simulink library "RealTimeLibrary"  (R2016b)
settings: Solver=ode45  StartTime=0.0  StopTime=10.0  RelTol=1e-3  EnableMultiTasking=on
undefined symbols (not defined in the file): CassieParameters, motor, pelvisMedulla
libraries: xpcethercatlib x75, simulink x1
settings Model: Creator=Mikhail  LastModifiedBy=Mikhail
settings DataIOCC: LimitDataPoints=on
settings OptimizationCC: LifeSpan=inf
settings DebuggingCC: AllowSymbolicDim=off  SFUnexpectedBacktrackingDiag=warning  SFNoUnconditionalDefaultTransitionDiag=warning  SFExecutionAtInitializationDiag=none
settings GRTTargetCC: TargetLangStandard=C89/C90 (ANSI)  GeneratePreprocessorConditionals=Disable all
settings ConfigComp: CovMetricSettings=dw  CovHtmlReporting=on  CovSaveCumulativeToWorkspaceVar=on  CovSaveSingleToWorkspaceVar=on  CovExternalEMLEnable=off

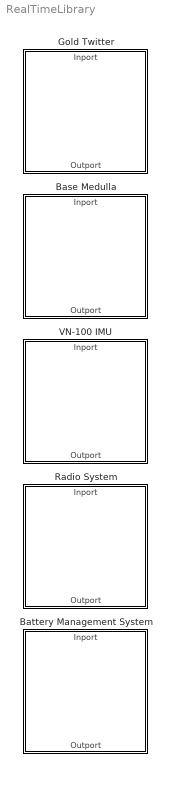
== system RealTimeLibrary ==
  Base Medulla : Subsystem  mask{structureName='pelvisMedulla', ethercatName='Pelvis Medulla'}
      mask prompts: structureName "Structure Name"; ethercatName "EtherCAT Name"
      mask init:
      | % Set bus assignments
      | set_param([gcb '/Base Inputs Bus Assignment'], ...
      |   'AssignedSignals', [...
      |     structureName '.baseInputs.cpuLoad,', ...
      |     structureName '.baseInputs.counter']);
      | 
      | % Set PDO recieve signal names
      | set_param([gcb '/CPU Load PDO Receive'], ...
      |   'sig_name', [ethercatName '.Base Inputs.CPU Load']);
      | set_param([gcb '/Counter PDO Receive'], ...
      |   'sig_name', [ethercatName '.Base Inputs.Counter']);
      mask Display: image('Medulla.png');
  Battery Management System : Subsystem
      mask Display: image('BQ76PL536A.png');
  Gold Twitter : Subsystem  mask{structureName='motor', ethercatName='Drive (Elmo Drive)', gearRatio=1, torqueConstant=1, encoderCounts=2^13, peakCurrentLimit=50}
      mask prompts: structureName "Structure Name"; ethercatName "EtherCAT Name"; gearRatio "Gear Ratio"; torqueConstant "Torque Constant"; encoderCounts "Encoder Counts"; peakCurrentLimit "Peak Current Limit"
      mask init:
      | % Set bus selectors
      | set_param([gcb '/Target Torque Bus Selector'], ...
      |   'OutputSignals', [structureName '.outputs.torque']);
      | set_param([gcb '/Status Word Bus Selector'], ...
      |   'OutputSignals', [structureName '.inputs.statusWord']);
      | 
      | % Set bus assignment
      | set_param([gcb '/Gold Twitter Bus Assignment'], ...
      |   'AssignedSignals', [...
      |     structureName '.inputs.statusWord,', ...
      |     structureName '.inputs.position,', ...
      |     structureName '.inputs.torque,', ...
      |     structureName '.inputs.amplifierTemperature,', ...
      |     structureName '.inputs.statorTemperature']);
      | 
      | % Set PDO transmit
      | set_param([gcb '/Mode of Operation PDO Transmit'], ...
      |   'sig_name', [ethercatName '.Outputs.Mode of operation']);
      | set_param([gcb '/Target Torque PDO Transmit'], ...
      |   'sig_name', [ethercatName '.Outputs.Target Torque']);
      | set_param([gcb '/Control Word PDO Transmit'], ...
      |   'sig_name', [ethercatName '.Outputs.Control word']);
      | 
      | % Set PDO receive
      | set_param([gcb '/Status Word PDO Receive'], ...
      |   'sig_name', [ethercatName '.Inputs.Status word']);
      | set_param([gcb '/Position PDO Receive'], ...
      |   'sig_name', [ethercatName '.Inputs.Position actual value']);
      | set_param([gcb '/Torque PDO Receive'], ...
      |   'sig_name', [ethercatName '.Inputs.Torque actual value']);
      | set_param([gcb '/Stator Temperature PDO Receive'], ...
      |   'sig_name', [ethercatName '.Inputs.Stator Temp']);
      | 
      | % Set SDO upload
      | set_param([gcb '/Amplifier Temperature Async SDO Upload'], ...
      |   'index', '8867');
      | set_param([gcb '/Amplifier Temperature Async SDO Upload'], ...
      |   'subIndex', '1');
      | set_param([gcb '/Amplifier Temperature Async SDO Upload'], ...
      |   'slave_name', ethercatName);
      mask Display: image('Gold Twitter.png')
  Radio System : Subsystem
      mask Display: image('Fr Sky Taranis.png');
  VN-100 IMU : Subsystem
      mask Display: image('VN-100 IMU.png');

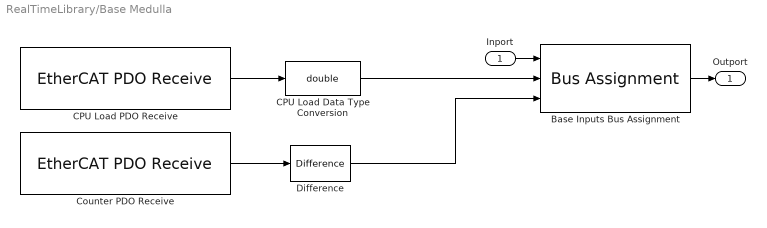
== system RealTimeLibrary/Base Medulla ==
  Inport : Inport  OutDataTypeStr=Bus: cassieEtherCATBus  SampleTime=CassieParameters.etherCATSampleTime
  Base Inputs Bus Assignment : BusAssignment  AssignedSignals=pelvisMedulla.baseInputs.cpuLoad,pelvisMedulla.baseInputs.counter
  CPU Load Data Type Conversion : DataTypeConversion  OutDataTypeStr=double
  CPU Load PDO Receive : xpcethercatlib/EtherCAT PDO Receive  Priority=2  sig_name=Pelvis Medulla.Base Inputs.CPU Load  sig_offset=600  sig_type=uint16  type_size=16  sig_dim=1  device_id=0  sample_time=0.000500
  Counter PDO Receive : xpcethercatlib/EtherCAT PDO Receive  Priority=2  sig_name=Pelvis Medulla.Base Inputs.Counter  sig_offset=592  sig_type=uint8  type_size=8  sig_dim=1  device_id=0  sample_time=0.000500
  Difference : simulink/Discrete/Difference  ICPrevInput=0.0  OutMin=[]  OutMax=[]  OutDataType=fixdt(1, 16)  OutScaling=2^-10  DoSatur=off
  Outport : Outport  OutDataTypeStr=Bus: cassieEtherCATBus  SampleTime=CassieParameters.etherCATSampleTime
  wires:
  Base Inputs Bus Assignment/1 -> Outport/1
  Counter PDO Receive/1 -> Difference/1
  Difference/1 -> Base Inputs Bus Assignment/3
  Inport/1 -> Base Inputs Bus Assignment/1
  CPU Load PDO Receive/1 -> CPU Load Data Type Conversion/1
  CPU Load Data Type Conversion/1 -> Base Inputs Bus Assignment/2

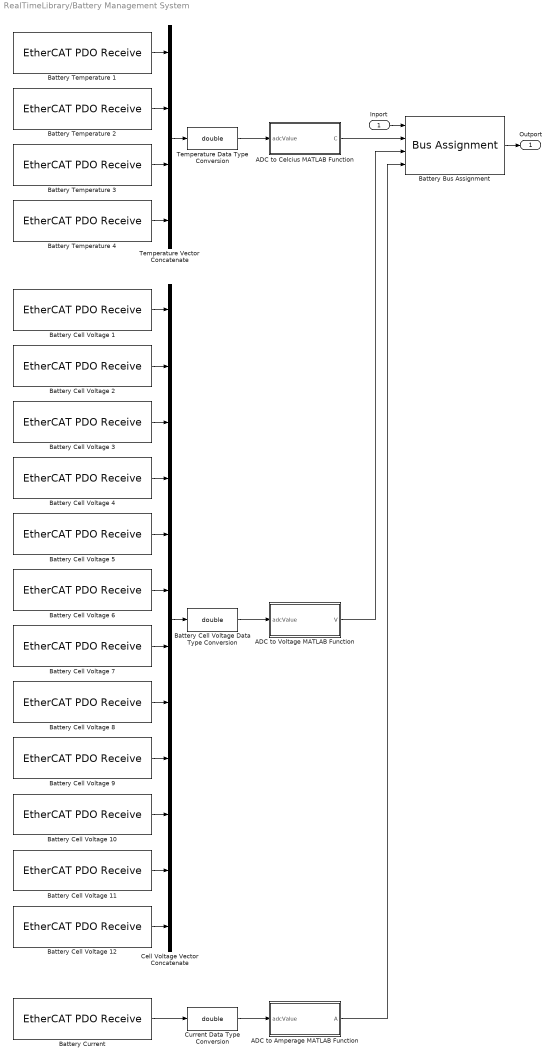
== system RealTimeLibrary/Battery Management System ==
  Inport : Inport  OutDataTypeStr=Bus: cassieEtherCATBus  SampleTime=CassieParameters.etherCATSampleTime
  ADC to Amperage MATLAB Function : MATLAB Function  TreatAsAtomicUnit=on
  ADC to Celcius MATLAB Function : MATLAB Function  TreatAsAtomicUnit=on
  ADC to Voltage MATLAB Function : MATLAB Function  TreatAsAtomicUnit=on
  Battery Bus Assignment : BusAssignment  AssignedSignals=pelvisMedulla.inputs.batteryTemperature,pelvisMedulla.inputs.batteryCellVoltage,pelvisMedulla.inputs.batteryCurrent
  Battery Cell Voltage Data Type Conversion : DataTypeConversion  OutDataTypeStr=double
  Battery Cell Voltage 1 : xpcethercatlib/EtherCAT PDO Receive  Priority=2  sig_name=Pelvis Medulla.BMS Inputs.Cell Voltage 01  sig_offset=1528  sig_type=uint16  type_size=16  sig_dim=1  device_id=0  sample_time=0.000500
  Battery Cell Voltage 10 : xpcethercatlib/EtherCAT PDO Receive  Priority=2  sig_name=Pelvis Medulla.BMS Inputs.Cell Voltage 10  sig_offset=1672  sig_type=uint16  type_size=16  sig_dim=1  device_id=0  sample_time=0.000500
  Battery Cell Voltage 11 : xpcethercatlib/EtherCAT PDO Receive  Priority=2  sig_name=Pelvis Medulla.BMS Inputs.Cell Voltage 11  sig_offset=1688  sig_type=uint16  type_size=16  sig_dim=1  device_id=0  sample_time=0.000500
  Battery Cell Voltage 12 : xpcethercatlib/EtherCAT PDO Receive  Priority=2  sig_name=Pelvis Medulla.BMS Inputs.Cell Voltage 12  sig_offset=1704  sig_type=uint16  type_size=16  sig_dim=1  device_id=0  sample_time=0.000500
  Battery Cell Voltage 2 : xpcethercatlib/EtherCAT PDO Receive  Priority=2  sig_name=Pelvis Medulla.BMS Inputs.Cell Voltage 02  sig_offset=1544  sig_type=uint16  type_size=16  sig_dim=1  device_id=0  sample_time=0.000500
  Battery Cell Voltage 3 : xpcethercatlib/EtherCAT PDO Receive  Priority=2  sig_name=Pelvis Medulla.BMS Inputs.Cell Voltage 03  sig_offset=1560  sig_type=uint16  type_size=16  sig_dim=1  device_id=0  sample_time=0.000500
  Battery Cell Voltage 4 : xpcethercatlib/EtherCAT PDO Receive  Priority=2  sig_name=Pelvis Medulla.BMS Inputs.Cell Voltage 04  sig_offset=1576  sig_type=uint16  type_size=16  sig_dim=1  device_id=0  sample_time=0.000500
  Battery Cell Voltage 5 : xpcethercatlib/EtherCAT PDO Receive  Priority=2  sig_name=Pelvis Medulla.BMS Inputs.Cell Voltage 05  sig_offset=1592  sig_type=uint16  type_size=16  sig_dim=1  device_id=0  sample_time=0.000500
  Battery Cell Voltage 6 : xpcethercatlib/EtherCAT PDO Receive  Priority=2  sig_name=Pelvis Medulla.BMS Inputs.Cell Voltage 06  sig_offset=1608  sig_type=uint16  type_size=16  sig_dim=1  device_id=0  sample_time=0.000500
  Battery Cell Voltage 7 : xpcethercatlib/EtherCAT PDO Receive  Priority=2  sig_name=Pelvis Medulla.BMS Inputs.Cell Voltage 07  sig_offset=1624  sig_type=uint16  type_size=16  sig_dim=1  device_id=0  sample_time=0.000500
  Battery Cell Voltage 8 : xpcethercatlib/EtherCAT PDO Receive  Priority=2  sig_name=Pelvis Medulla.BMS Inputs.Cell Voltage 08  sig_offset=1640  sig_type=uint16  type_size=16  sig_dim=1  device_id=0  sample_time=0.000500
  Battery Cell Voltage 9 : xpcethercatlib/EtherCAT PDO Receive  Priority=2  sig_name=Pelvis Medulla.BMS Inputs.Cell Voltage 09  sig_offset=1656  sig_type=uint16  type_size=16  sig_dim=1  device_id=0  sample_time=0.000500
  Battery Current : xpcethercatlib/EtherCAT PDO Receive  Priority=2  sig_name=Pelvis Medulla.BMS Inputs.Current  sig_offset=1784  sig_type=uint16  type_size=16  sig_dim=1  device_id=0  sample_time=0.000500
  Battery Temperature 1 : xpcethercatlib/EtherCAT PDO Receive  Priority=2  sig_name=Pelvis Medulla.BMS Inputs.Temperature 1  sig_offset=1720  sig_type=uint16  type_size=16  sig_dim=1  device_id=0  sample_time=0.000500
  Battery Temperature 2 : xpcethercatlib/EtherCAT PDO Receive  Priority=2  sig_name=Pelvis Medulla.BMS Inputs.Temperature 2  sig_offset=1736  sig_type=uint16  type_size=16  sig_dim=1  device_id=0  sample_time=0.000500
  Battery Temperature 3 : xpcethercatlib/EtherCAT PDO Receive  Priority=2  sig_name=Pelvis Medulla.BMS Inputs.Temperature 3  sig_offset=1752  sig_type=uint16  type_size=16  sig_dim=1  device_id=0  sample_time=0.000500
  Battery Temperature 4 : xpcethercatlib/EtherCAT PDO Receive  Priority=2  sig_name=Pelvis Medulla.BMS Inputs.Temperature 4  sig_offset=1768  sig_type=uint16  type_size=16  sig_dim=1  device_id=0  sample_time=0.000500
  Cell Voltage Vector Concatenate : Concatenate  NumInputs=12
  Current Data Type Conversion : DataTypeConversion  OutDataTypeStr=double
  Temperature Data Type Conversion : DataTypeConversion  OutDataTypeStr=double
  Temperature Vector Concatenate : Concatenate  NumInputs=4
  Outport : Outport  OutDataTypeStr=Bus: cassieEtherCATBus  SampleTime=CassieParameters.etherCATSampleTime
  wires:
  Battery Temperature 1/1 -> Temperature Vector Concatenate/1
  Battery Temperature 2/1 -> Temperature Vector Concatenate/2
  Battery Temperature 3/1 -> Temperature Vector Concatenate/3
  Battery Temperature 4/1 -> Temperature Vector Concatenate/4
  Battery Cell Voltage 1/1 -> Cell Voltage Vector Concatenate/1
  Battery Cell Voltage 2/1 -> Cell Voltage Vector Concatenate/2
  Battery Cell Voltage 3/1 -> Cell Voltage Vector Concatenate/3
  Battery Cell Voltage 4/1 -> Cell Voltage Vector Concatenate/4
  Battery Cell Voltage 5/1 -> Cell Voltage Vector Concatenate/5
  Battery Cell Voltage 6/1 -> Cell Voltage Vector Concatenate/6
  Battery Cell Voltage 7/1 -> Cell Voltage Vector Concatenate/7
  Battery Cell Voltage 8/1 -> Cell Voltage Vector Concatenate/8
  Battery Cell Voltage 9/1 -> Cell Voltage Vector Concatenate/9
  Battery Cell Voltage 10/1 -> Cell Voltage Vector Concatenate/10
  Battery Cell Voltage 11/1 -> Cell Voltage Vector Concatenate/11
  Battery Cell Voltage 12/1 -> Cell Voltage Vector Concatenate/12
  Temperature Vector Concatenate/1 -> Temperature Data Type Conversion/1
  Cell Voltage Vector Concatenate/1 -> Battery Cell Voltage Data Type Conversion/1
  ADC to Voltage MATLAB Function/1(V) -> Battery Bus Assignment/3
  Battery Current/1 -> Current Data Type Conversion/1
  ADC to Celcius MATLAB Function/1(C) -> Battery Bus Assignment/2
  Battery Bus Assignment/1 -> Outport/1
  Inport/1 -> Battery Bus Assignment/1
  Temperature Data Type Conversion/1 -> ADC to Celcius MATLAB Function/1(adcValue)
  Battery Cell Voltage Data Type Conversion/1 -> ADC to Voltage MATLAB Function/1(adcValue)
  ADC to Amperage MATLAB Function/1(A) -> Battery Bus Assignment/4
  Current Data Type Conversion/1 -> ADC to Amperage MATLAB Function/1(adcValue)

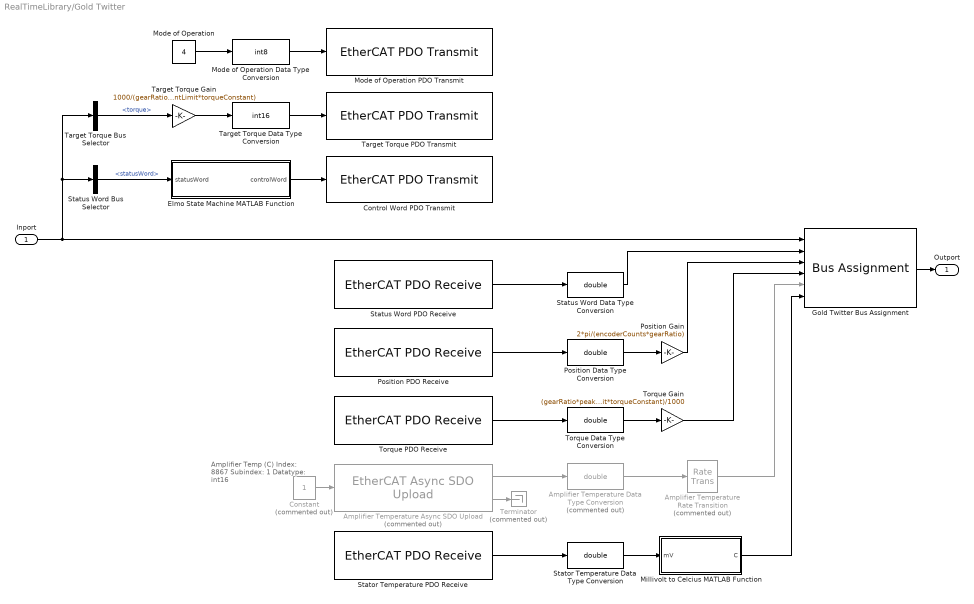
== system RealTimeLibrary/Gold Twitter ==
  note: Amplifier Temp (C)
      | Index: 8867
      | Subindex: 1
      | Datatype: int16
  Inport : Inport  PortDimensions=1
  Amplifier Temperature Data Type Conversion : DataTypeConversion  Commented=on  OutDataTypeStr=double
  Amplifier Temperature Rate Transition : RateTransition  Commented=on
  Amplifier Temperature Async SDO Upload : xpcethercatlib/EtherCAT Async SDO Upload  Commented=on  index=8867  subIndex=1  sig_type=int16  sig_dim=1  device_id=0  slave_name=Drive (Elmo Drive)  sample_time=1/100  slave_addr=0  selected_slave=Term 1 (EK1100)  timeout=500  slave_found=0
  Constant : Constant  Commented=on  OutDataTypeStr=int32
  Control Word PDO Transmit : xpcethercatlib/EtherCAT PDO Transmit   Priority=3  sig_name=Drive (Elmo Drive).Outputs.Control word  sig_offset=2144  sig_type=uint16  type_size=16  sig_dim=1  device_id=0  sample_time=0.001000
  Elmo State Machine MATLAB Function : MATLAB Function  TreatAsAtomicUnit=on
  Gold Twitter Bus Assignment : BusAssignment  AssignedSignals=motor.inputs.statusWord,motor.inputs.position,motor.inputs.torque,motor.inputs.amplifierTemperature,motor.inputs.statorTemperature
  Millivolt to Celcius MATLAB Function : MATLAB Function  TreatAsAtomicUnit=on
  Mode of Operation : Constant  Value=4  OutDataTypeStr=Inherit: Inherit via back propagation
  Mode of Operation Data Type Conversion : DataTypeConversion  OutDataTypeStr=int8
  Mode of Operation PDO Transmit : xpcethercatlib/EtherCAT PDO Transmit   Priority=3  sig_name=Drive (Elmo Drive).Outputs.Mode of operation  sig_offset=2160  sig_type=int8  type_size=8  sig_dim=1  device_id=0  sample_time=0.001000
  Position Data Type Conversion : DataTypeConversion  OutDataTypeStr=double
  Position Gain : Gain  Gain=2*pi/(encoderCounts*gearRatio)
  Position PDO Receive : xpcethercatlib/EtherCAT PDO Receive  Priority=2  sig_name=Drive (Elmo Drive).Inputs.Position actual value  sig_offset=2128  sig_type=int32  type_size=32  sig_dim=1  device_id=0  sample_time=0.001000
  Stator Temperature Data Type Conversion : DataTypeConversion  OutDataTypeStr=double
  Stator Temperature PDO Receive : xpcethercatlib/EtherCAT PDO Receive  Priority=2  sig_name=Drive (Elmo Drive).Inputs.Stator Temp  sig_offset=2128  sig_type=int32  type_size=32  sig_dim=1  device_id=0  sample_time=0.001000
  Status Word Bus Selector : BusSelector  OutputSignals=motor.inputs.statusWord
  Status Word Data Type Conversion : DataTypeConversion  OutDataTypeStr=double
  Status Word PDO Receive : xpcethercatlib/EtherCAT PDO Receive  Priority=2  sig_name=Drive (Elmo Drive).Inputs.Status word  sig_offset=2176  sig_type=uint16  type_size=16  sig_dim=1  device_id=0  sample_time=0.001000
  Target Torque Bus Selector : BusSelector  OutputSignals=motor.outputs.torque
  Target Torque Data Type Conversion : DataTypeConversion  OutDataTypeStr=int16
  Target Torque Gain : Gain  Gain=1000/(gearRatio*peakCurrentLimit*torqueConstant)
  Target Torque PDO Transmit : xpcethercatlib/EtherCAT PDO Transmit   Priority=3  sig_name=Drive (Elmo Drive).Outputs.Target Torque  sig_offset=2128  sig_type=int16  type_size=16  sig_dim=1  device_id=0  sample_time=0.001000
  Terminator : Terminator  Commented=on
  Torque Data Type Conversion : DataTypeConversion  OutDataTypeStr=double
  Torque Gain : Gain  Gain=(gearRatio*peakCurrentLimit*torqueConstant)/1000
  Torque PDO Receive : xpcethercatlib/EtherCAT PDO Receive  Priority=2  sig_name=Drive (Elmo Drive).Inputs.Torque actual value  sig_offset=2128  sig_type=int32  type_size=32  sig_dim=1  device_id=0  sample_time=0.001000
  Outport : Outport  PortDimensions=1
  wires:
  Status Word Data Type Conversion/1 -> Gold Twitter Bus Assignment/2
  Position Data Type Conversion/1 -> Position Gain/1
  Target Torque Bus Selector/1 -> Target Torque Gain/1  "<torque>"
  Gold Twitter Bus Assignment/1 -> Outport/1
  Target Torque Gain/1 -> Target Torque Data Type Conversion/1
  Position PDO Receive/1 -> Position Data Type Conversion/1
  Target Torque Data Type Conversion/1 -> Target Torque PDO Transmit/1
  Mode of Operation Data Type Conversion/1 -> Mode of Operation PDO Transmit/1
  Mode of Operation/1 -> Mode of Operation Data Type Conversion/1
  Status Word PDO Receive/1 -> Status Word Data Type Conversion/1
  Elmo State Machine MATLAB Function/1(controlWord) -> Control Word PDO Transmit/1
  Inport/1 -> Status Word Bus Selector/1, Target Torque Bus Selector/1, Gold Twitter Bus Assignment/1
  Status Word Bus Selector/1 -> Elmo State Machine MATLAB Function/1(statusWord)  "<statusWord>"
  Torque Data Type Conversion/1 -> Torque Gain/1
  Torque PDO Receive/1 -> Torque Data Type Conversion/1
  Position Gain/1 -> Gold Twitter Bus Assignment/3
  Torque Gain/1 -> Gold Twitter Bus Assignment/4
  Constant/1 -> Amplifier Temperature Async SDO Upload/1
  Amplifier Temperature Async SDO Upload/1 -> Amplifier Temperature Data Type Conversion/1
  Amplifier Temperature Async SDO Upload/2 -> Terminator/1
  Stator Temperature Data Type Conversion/1 -> Millivolt to Celcius MATLAB Function/1(mV)
  Stator Temperature PDO Receive/1 -> Stator Temperature Data Type Conversion/1
  Amplifier Temperature Data Type Conversion/1 -> Amplifier Temperature Rate Transition/1
  Millivolt to Celcius MATLAB Function/1(C) -> Gold Twitter Bus Assignment/6
  Amplifier Temperature Rate Transition/1 -> Gold Twitter Bus Assignment/5

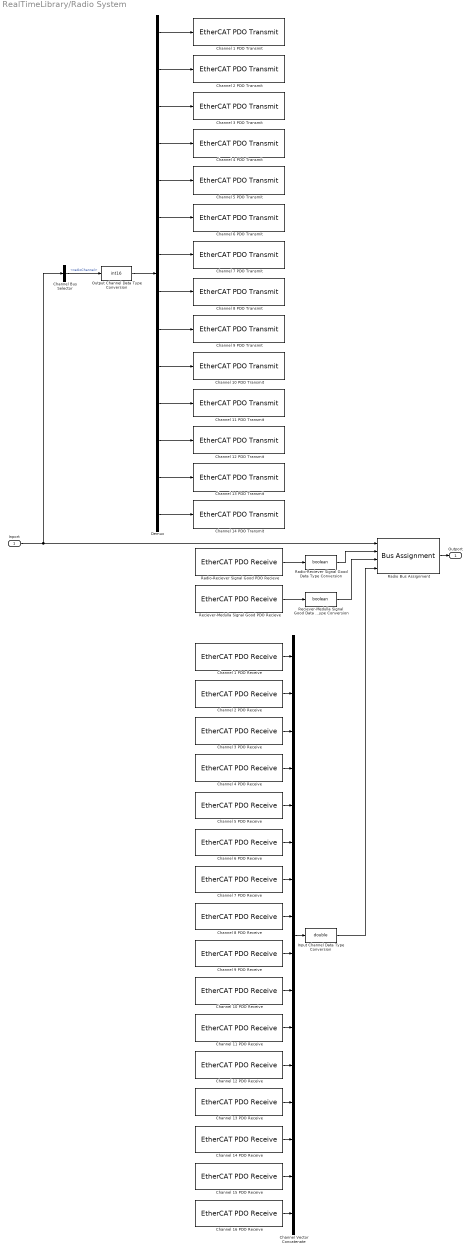
== system RealTimeLibrary/Radio System ==
  Inport : Inport  OutDataTypeStr=Bus: cassieEtherCATBus  SampleTime=CassieParameters.etherCATSampleTime
  Channel Bus Selector : BusSelector  OutputSignals=pelvisMedulla.outputs.radioChannel
  Channel Vector Concatenate : Concatenate  NumInputs=16
  Channel 1 PDO Receive : xpcethercatlib/EtherCAT PDO Receive  Priority=2  sig_name=Pelvis Medulla.Radio Inputs.Channel 01  sig_offset=616  sig_type=int16  type_size=16  sig_dim=1  device_id=0  sample_time=0.000500
  Channel 1 PDO Transmit : xpcethercatlib/EtherCAT PDO Transmit   Priority=3  sig_name=Pelvis Medulla.Radio Outputs.Channel 01  sig_offset=592  sig_type=int16  type_size=16  sig_dim=1  device_id=0  sample_time=0.000500
  Channel 10 PDO Receive : xpcethercatlib/EtherCAT PDO Receive  Priority=2  sig_name=Pelvis Medulla.Radio Inputs.Channel 10  sig_offset=760  sig_type=int16  type_size=16  sig_dim=1  device_id=0  sample_time=0.000500
  Channel 10 PDO Transmit : xpcethercatlib/EtherCAT PDO Transmit   Priority=3  sig_name=Pelvis Medulla.Radio Outputs.Channel 10  sig_offset=736  sig_type=int16  type_size=16  sig_dim=1  device_id=0  sample_time=0.000500
  Channel 11 PDO Receive : xpcethercatlib/EtherCAT PDO Receive  Priority=2  sig_name=Pelvis Medulla.Radio Inputs.Channel 11  sig_offset=776  sig_type=int16  type_size=16  sig_dim=1  device_id=0  sample_time=0.000500
  Channel 11 PDO Transmit : xpcethercatlib/EtherCAT PDO Transmit   Priority=3  sig_name=Pelvis Medulla.Radio Outputs.Channel 11  sig_offset=752  sig_type=int16  type_size=16  sig_dim=1  device_id=0  sample_time=0.000500
  Channel 12 PDO Receive : xpcethercatlib/EtherCAT PDO Receive  Priority=2  sig_name=Pelvis Medulla.Radio Inputs.Channel 12  sig_offset=792  sig_type=int16  type_size=16  sig_dim=1  device_id=0  sample_time=0.000500
  Channel 12 PDO Transmit : xpcethercatlib/EtherCAT PDO Transmit   Priority=3  sig_name=Pelvis Medulla.Radio Outputs.Channel 12  sig_offset=768  sig_type=int16  type_size=16  sig_dim=1  device_id=0  sample_time=0.000500
  Channel 13 PDO Receive : xpcethercatlib/EtherCAT PDO Receive  Priority=2  sig_name=Pelvis Medulla.Radio Inputs.Channel 13  sig_offset=808  sig_type=int16  type_size=16  sig_dim=1  device_id=0  sample_time=0.000500
  Channel 13 PDO Transmit : xpcethercatlib/EtherCAT PDO Transmit   Priority=3  sig_name=Pelvis Medulla.Radio Outputs.Channel 13  sig_offset=784  sig_type=int16  type_size=16  sig_dim=1  device_id=0  sample_time=0.000500
  Channel 14 PDO Receive : xpcethercatlib/EtherCAT PDO Receive  Priority=2  sig_name=Pelvis Medulla.Radio Inputs.Channel 14  sig_offset=824  sig_type=int16  type_size=16  sig_dim=1  device_id=0  sample_time=0.000500
  Channel 14 PDO Transmit : xpcethercatlib/EtherCAT PDO Transmit   Priority=3  sig_name=Pelvis Medulla.Radio Outputs.Channel 14  sig_offset=800  sig_type=int16  type_size=16  sig_dim=1  device_id=0  sample_time=0.000500
  Channel 15 PDO Receive : xpcethercatlib/EtherCAT PDO Receive  Priority=2  sig_name=Pelvis Medulla.Radio Inputs.Channel 15  sig_offset=840  sig_type=int16  type_size=16  sig_dim=1  device_id=0  sample_time=0.000500
  Channel 16 PDO Receive : xpcethercatlib/EtherCAT PDO Receive  Priority=2  sig_name=Pelvis Medulla.Radio Inputs.Channel 16  sig_offset=856  sig_type=int16  type_size=16  sig_dim=1  device_id=0  sample_time=0.000500
  Channel 2 PDO Receive : xpcethercatlib/EtherCAT PDO Receive  Priority=2  sig_name=Pelvis Medulla.Radio Inputs.Channel 02  sig_offset=632  sig_type=int16  type_size=16  sig_dim=1  device_id=0  sample_time=0.000500
  Channel 2 PDO Transmit : xpcethercatlib/EtherCAT PDO Transmit   Priority=3  sig_name=Pelvis Medulla.Radio Outputs.Channel 02  sig_offset=608  sig_type=int16  type_size=16  sig_dim=1  device_id=0  sample_time=0.000500
  Channel 3 PDO Receive : xpcethercatlib/EtherCAT PDO Receive  Priority=2  sig_name=Pelvis Medulla.Radio Inputs.Channel 03  sig_offset=648  sig_type=int16  type_size=16  sig_dim=1  device_id=0  sample_time=0.000500
  Channel 3 PDO Transmit : xpcethercatlib/EtherCAT PDO Transmit   Priority=3  sig_name=Pelvis Medulla.Radio Outputs.Channel 03  sig_offset=624  sig_type=int16  type_size=16  sig_dim=1  device_id=0  sample_time=0.000500
  Channel 4 PDO Receive : xpcethercatlib/EtherCAT PDO Receive  Priority=2  sig_name=Pelvis Medulla.Radio Inputs.Channel 04  sig_offset=664  sig_type=int16  type_size=16  sig_dim=1  device_id=0  sample_time=0.000500
  Channel 4 PDO Transmit : xpcethercatlib/EtherCAT PDO Transmit   Priority=3  sig_name=Pelvis Medulla.Radio Outputs.Channel 04  sig_offset=640  sig_type=int16  type_size=16  sig_dim=1  device_id=0  sample_time=0.000500
  Channel 5 PDO Receive : xpcethercatlib/EtherCAT PDO Receive  Priority=2  sig_name=Pelvis Medulla.Radio Inputs.Channel 05  sig_offset=680  sig_type=int16  type_size=16  sig_dim=1  device_id=0  sample_time=0.000500
  Channel 5 PDO Transmit : xpcethercatlib/EtherCAT PDO Transmit   Priority=3  sig_name=Pelvis Medulla.Radio Outputs.Channel 05  sig_offset=656  sig_type=int16  type_size=16  sig_dim=1  device_id=0  sample_time=0.000500
  Channel 6 PDO Receive : xpcethercatlib/EtherCAT PDO Receive  Priority=2  sig_name=Pelvis Medulla.Radio Inputs.Channel 06  sig_offset=696  sig_type=int16  type_size=16  sig_dim=1  device_id=0  sample_time=0.000500
  Channel 6 PDO Transmit : xpcethercatlib/EtherCAT PDO Transmit   Priority=3  sig_name=Pelvis Medulla.Radio Outputs.Channel 06  sig_offset=672  sig_type=int16  type_size=16  sig_dim=1  device_id=0  sample_time=0.000500
  Channel 7 PDO Receive : xpcethercatlib/EtherCAT PDO Receive  Priority=2  sig_name=Pelvis Medulla.Radio Inputs.Channel 07  sig_offset=712  sig_type=int16  type_size=16  sig_dim=1  device_id=0  sample_time=0.000500
  Channel 7 PDO Transmit : xpcethercatlib/EtherCAT PDO Transmit   Priority=3  sig_name=Pelvis Medulla.Radio Outputs.Channel 07  sig_offset=688  sig_type=int16  type_size=16  sig_dim=1  device_id=0  sample_time=0.000500
  Channel 8 PDO Receive : xpcethercatlib/EtherCAT PDO Receive  Priority=2  sig_name=Pelvis Medulla.Radio Inputs.Channel 08  sig_offset=728  sig_type=int16  type_size=16  sig_dim=1  device_id=0  sample_time=0.000500
  Channel 8 PDO Transmit : xpcethercatlib/EtherCAT PDO Transmit   Priority=3  sig_name=Pelvis Medulla.Radio Outputs.Channel 08  sig_offset=704  sig_type=int16  type_size=16  sig_dim=1  device_id=0  sample_time=0.000500
  Channel 9 PDO Receive : xpcethercatlib/EtherCAT PDO Receive  Priority=2  sig_name=Pelvis Medulla.Radio Inputs.Channel 09  sig_offset=744  sig_type=int16  type_size=16  sig_dim=1  device_id=0  sample_time=0.000500
  Channel 9 PDO Transmit : xpcethercatlib/EtherCAT PDO Transmit   Priority=3  sig_name=Pelvis Medulla.Radio Outputs.Channel 09  sig_offset=720  sig_type=int16  type_size=16  sig_dim=1  device_id=0  sample_time=0.000500
  Demux : Demux  Outputs=14
  Input Channel Data Type Conversion : DataTypeConversion  OutDataTypeStr=double
  Output Channel Data Type Conversion : DataTypeConversion  OutDataTypeStr=int16
  Radio Bus Assignment : BusAssignment  AssignedSignals=pelvisMedulla.inputs.radioRecieverSignalGood,pelvisMedulla.inputs.recieverMedullaSignalGood,pelvisMedulla.inputs.radioChannel
  Radio-Reciever Signal Good Data Type Conversion : DataTypeConversion  OutDataTypeStr=boolean
  Radio-Reciever Signal Good PDO Recieve : xpcethercatlib/EtherCAT PDO Receive  Priority=2  sig_name=Pelvis Medulla.Status Inputs.Radio-Receiver Signal Good  sig_offset=1805  sig_type=boolean  type_size=1  sig_dim=1  device_id=0  sample_time=0.000500
  Reciever-Medulla Signal Good Data Type Conversion : DataTypeConversion  OutDataTypeStr=boolean
  Reciever-Medulla Signal Good PDO Recieve : xpcethercatlib/EtherCAT PDO Receive  Priority=2  sig_name=Pelvis Medulla.Status Inputs.Receiver-Medulla Signal Good  sig_offset=1806  sig_type=boolean  type_size=1  sig_dim=1  device_id=0  sample_time=0.000500
  Outport : Outport  OutDataTypeStr=Bus: cassieEtherCATBus  SampleTime=CassieParameters.etherCATSampleTime
  wires:
  Radio Bus Assignment/1 -> Outport/1
  Channel 1 PDO Receive/1 -> Channel Vector Concatenate/1
  Channel 2 PDO Receive/1 -> Channel Vector Concatenate/2
  Channel 16 PDO Receive/1 -> Channel Vector Concatenate/16
  Channel 15 PDO Receive/1 -> Channel Vector Concatenate/15
  Channel 14 PDO Receive/1 -> Channel Vector Concatenate/14
  Channel 13 PDO Receive/1 -> Channel Vector Concatenate/13
  Channel 12 PDO Receive/1 -> Channel Vector Concatenate/12
  Channel 11 PDO Receive/1 -> Channel Vector Concatenate/11
  Channel 10 PDO Receive/1 -> Channel Vector Concatenate/10
  Channel 9 PDO Receive/1 -> Channel Vector Concatenate/9
  Channel 8 PDO Receive/1 -> Channel Vector Concatenate/8
  Channel 6 PDO Receive/1 -> Channel Vector Concatenate/6
  Channel 7 PDO Receive/1 -> Channel Vector Concatenate/7
  Channel 3 PDO Receive/1 -> Channel Vector Concatenate/3
  Channel 4 PDO Receive/1 -> Channel Vector Concatenate/4
  Channel 5 PDO Receive/1 -> Channel Vector Concatenate/5
  Channel Vector Concatenate/1 -> Input Channel Data Type Conversion/1
  Input Channel Data Type Conversion/1 -> Radio Bus Assignment/4
  Reciever-Medulla Signal Good PDO Recieve/1 -> Reciever-Medulla Signal Good Data Type Conversion/1
  Radio-Reciever Signal Good PDO Recieve/1 -> Radio-Reciever Signal Good Data Type Conversion/1
  Reciever-Medulla Signal Good Data Type Conversion/1 -> Radio Bus Assignment/3
  Radio-Reciever Signal Good Data Type Conversion/1 -> Radio Bus Assignment/2
  Channel Bus Selector/1 -> Output Channel Data Type Conversion/1  "<radioChannel>"
  Inport/1 -> Channel Bus Selector/1, Radio Bus Assignment/1
  Demux/1 -> Channel 1 PDO Transmit/1
  Demux/14 -> Channel 14 PDO Transmit/1
  Demux/2 -> Channel 2 PDO Transmit/1
  Demux/3 -> Channel 3 PDO Transmit/1
  Demux/4 -> Channel 4 PDO Transmit/1
  Demux/5 -> Channel 5 PDO Transmit/1
  Demux/6 -> Channel 6 PDO Transmit/1
  Demux/7 -> Channel 7 PDO Transmit/1
  Demux/8 -> Channel 8 PDO Transmit/1
  Demux/9 -> Channel 9 PDO Transmit/1
  Demux/10 -> Channel 10 PDO Transmit/1
  Demux/11 -> Channel 11 PDO Transmit/1
  Demux/12 -> Channel 12 PDO Transmit/1
  Demux/13 -> Channel 13 PDO Transmit/1
  Output Channel Data Type Conversion/1 -> Demux/1

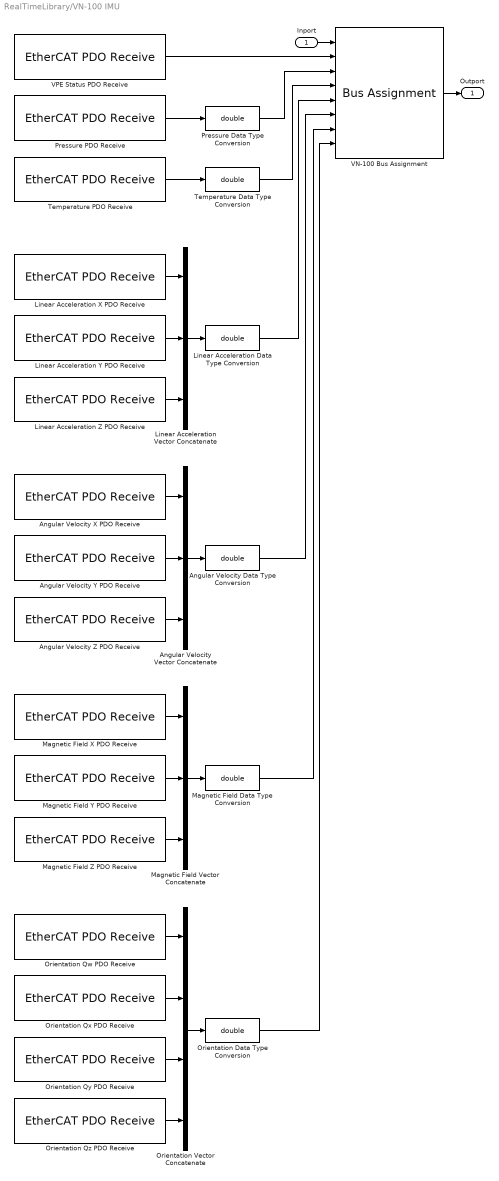
== system RealTimeLibrary/VN-100 IMU ==
  Inport : Inport  OutDataTypeStr=Bus: cassieEtherCATBus  SampleTime=CassieParameters.etherCATSampleTime
  Angular Velocity Data Type Conversion : DataTypeConversion  OutDataTypeStr=double
  Angular Velocity Vector Concatenate : Concatenate  NumInputs=3
  Angular Velocity X PDO Receive : xpcethercatlib/EtherCAT PDO Receive  Priority=2  sig_name=Pelvis Medulla.VN Inputs.Angular Velocity X  sig_offset=1160  sig_type=single  type_size=32  sig_dim=1  device_id=0  sample_time=0.000500
  Angular Velocity Y PDO Receive : xpcethercatlib/EtherCAT PDO Receive  Priority=2  sig_name=Pelvis Medulla.VN Inputs.Angular Velocity Y  sig_offset=1192  sig_type=single  type_size=32  sig_dim=1  device_id=0  sample_time=0.000500
  Angular Velocity Z PDO Receive : xpcethercatlib/EtherCAT PDO Receive  Priority=2  sig_name=Pelvis Medulla.VN Inputs.Angular Velocity Z  sig_offset=1224  sig_type=single  type_size=32  sig_dim=1  device_id=0  sample_time=0.000500
  Linear Acceleration Data Type Conversion : DataTypeConversion  OutDataTypeStr=double
  Linear Acceleration Vector Concatenate : Concatenate  NumInputs=3
  Linear Acceleration X PDO Receive : xpcethercatlib/EtherCAT PDO Receive  Priority=2  sig_name=Pelvis Medulla.VN Inputs.Linear Acceleration X  sig_offset=1256  sig_type=single  type_size=32  sig_dim=1  device_id=0  sample_time=0.000500
  Linear Acceleration Y PDO Receive : xpcethercatlib/EtherCAT PDO Receive  Priority=2  sig_name=Pelvis Medulla.VN Inputs.Linear Acceleration Y  sig_offset=1288  sig_type=single  type_size=32  sig_dim=1  device_id=0  sample_time=0.000500
  Linear Acceleration Z PDO Receive : xpcethercatlib/EtherCAT PDO Receive  Priority=2  sig_name=Pelvis Medulla.VN Inputs.Linear Acceleration Z  sig_offset=1320  sig_type=single  type_size=32  sig_dim=1  device_id=0  sample_time=0.000500
  Magnetic Field Data Type Conversion : DataTypeConversion  OutDataTypeStr=double
  Magnetic Field Vector Concatenate : Concatenate  NumInputs=3
  Magnetic Field X PDO Receive : xpcethercatlib/EtherCAT PDO Receive  Priority=2  sig_name=Pelvis Medulla.VN Inputs.Magnetic Field X  sig_offset=1352  sig_type=single  type_size=32  sig_dim=1  device_id=0  sample_time=0.000500
  Magnetic Field Y PDO Receive : xpcethercatlib/EtherCAT PDO Receive  Priority=2  sig_name=Pelvis Medulla.VN Inputs.Magnetic Field Y  sig_offset=1384  sig_type=single  type_size=32  sig_dim=1  device_id=0  sample_time=0.000500
  Magnetic Field Z PDO Receive : xpcethercatlib/EtherCAT PDO Receive  Priority=2  sig_name=Pelvis Medulla.VN Inputs.Magnetic Field Z  sig_offset=1416  sig_type=single  type_size=32  sig_dim=1  device_id=0  sample_time=0.000500
  Orientation Data Type Conversion : DataTypeConversion  OutDataTypeStr=double
  Orientation Vector Concatenate : Concatenate  NumInputs=4
  Orientation Qw PDO Receive : xpcethercatlib/EtherCAT PDO Receive  Priority=2  sig_name=Pelvis Medulla.VN Inputs.Orientation Qw  sig_offset=1128  sig_type=single  type_size=32  sig_dim=1  device_id=0  sample_time=0.000500
  Orientation Qx PDO Receive : xpcethercatlib/EtherCAT PDO Receive  Priority=2  sig_name=Pelvis Medulla.VN Inputs.Orientation Qx  sig_offset=1032  sig_type=single  type_size=32  sig_dim=1  device_id=0  sample_time=0.000500
  Orientation Qy PDO Receive : xpcethercatlib/EtherCAT PDO Receive  Priority=2  sig_name=Pelvis Medulla.VN Inputs.Orientation Qy  sig_offset=1064  sig_type=single  type_size=32  sig_dim=1  device_id=0  sample_time=0.000500
  Orientation Qz PDO Receive : xpcethercatlib/EtherCAT PDO Receive  Priority=2  sig_name=Pelvis Medulla.VN Inputs.Orientation Qz  sig_offset=1096  sig_type=single  type_size=32  sig_dim=1  device_id=0  sample_time=0.000500
  Pressure Data Type Conversion : DataTypeConversion  OutDataTypeStr=double
  Pressure PDO Receive : xpcethercatlib/EtherCAT PDO Receive  Priority=2  sig_name=Pelvis Medulla.VN Inputs.Pressure  sig_offset=1480  sig_type=single  type_size=32  sig_dim=1  device_id=0  sample_time=0.000500
  Temperature Data Type Conversion : DataTypeConversion  OutDataTypeStr=double
  Temperature PDO Receive : xpcethercatlib/EtherCAT PDO Receive  Priority=2  sig_name=Pelvis Medulla.VN Inputs.Temperature  sig_offset=1448  sig_type=single  type_size=32  sig_dim=1  device_id=0  sample_time=0.000500
  VN-100 Bus Assignment : BusAssignment  AssignedSignals=pelvisMedulla.inputs.vnVPEStatus,pelvisMedulla.inputs.vnPressure,pelvisMedulla.inputs.vnTemperature,pelvisMedulla.inputs.vnLinearAcceleration,pelvisMedulla.inputs.vnAngularVelocity,pelvisMedulla.inputs.vnMagneticField,pelvisMedulla.inputs.vnOrientation
  VPE Status PDO Receive : xpcethercatlib/EtherCAT PDO Receive  Priority=2  sig_name=Pelvis Medulla.VN Inputs.VPE Status  sig_offset=1512  sig_type=uint16  type_size=16  sig_dim=1  device_id=0  sample_time=0.000500
  Outport : Outport  OutDataTypeStr=Bus: cassieEtherCATBus  SampleTime=CassieParameters.etherCATSampleTime
  wires:
  VN-100 Bus Assignment/1 -> Outport/1
  Temperature PDO Receive/1 -> Temperature Data Type Conversion/1
  Temperature Data Type Conversion/1 -> VN-100 Bus Assignment/4
  Pressure PDO Receive/1 -> Pressure Data Type Conversion/1
  Pressure Data Type Conversion/1 -> VN-100 Bus Assignment/3
  Inport/1 -> VN-100 Bus Assignment/1
  Linear Acceleration Vector Concatenate/1 -> Linear Acceleration Data Type Conversion/1
  Angular Velocity Vector Concatenate/1 -> Angular Velocity Data Type Conversion/1
  Linear Acceleration Y PDO Receive/1 -> Linear Acceleration Vector Concatenate/2
  Angular Velocity Y PDO Receive/1 -> Angular Velocity Vector Concatenate/2
  Linear Acceleration X PDO Receive/1 -> Linear Acceleration Vector Concatenate/1
  Linear Acceleration Z PDO Receive/1 -> Linear Acceleration Vector Concatenate/3
  Angular Velocity X PDO Receive/1 -> Angular Velocity Vector Concatenate/1
  Angular Velocity Z PDO Receive/1 -> Angular Velocity Vector Concatenate/3
  Angular Velocity Data Type Conversion/1 -> VN-100 Bus Assignment/6
  Linear Acceleration Data Type Conversion/1 -> VN-100 Bus Assignment/5
  Orientation Vector Concatenate/1 -> Orientation Data Type Conversion/1
  Orientation Qx PDO Receive/1 -> Orientation Vector Concatenate/2
  Orientation Qw PDO Receive/1 -> Orientation Vector Concatenate/1
  Orientation Qy PDO Receive/1 -> Orientation Vector Concatenate/3
  Orientation Qz PDO Receive/1 -> Orientation Vector Concatenate/4
  Orientation Data Type Conversion/1 -> VN-100 Bus Assignment/8
  Magnetic Field Vector Concatenate/1 -> Magnetic Field Data Type Conversion/1
  Magnetic Field Y PDO Receive/1 -> Magnetic Field Vector Concatenate/2
  Magnetic Field X PDO Receive/1 -> Magnetic Field Vector Concatenate/1
  Magnetic Field Z PDO Receive/1 -> Magnetic Field Vector Concatenate/3
  Magnetic Field Data Type Conversion/1 -> VN-100 Bus Assignment/7
  VPE Status PDO Receive/1 -> VN-100 Bus Assignment/2

== matlab function RealTimeLibrary/Gold Twitter/Elmo State Machine MATLAB Function ==
  data: statusWord input; controlWord output
function controlWord = elmoStateMachine(statusWord) %#codegen
%ELMOSTATEMACHINE Elmo amplifier state machine.
%
% Control Word (uint16) (Pg. 27 DSP 402):
%   0 - Switch on (M)
%   1 - Enable voltage (M)
%   2 - Quick stop (M)
%   3 - Enable operation (M)
%   4...6 - Operation mode specific (O)
%   7 - Fault reset (M)
%   8 - Hault (O)
%   9...10 - Reserved (O)
%   11...15 - Manufacturer specific (O)
% 
% Control commands (Bits 0,1,2,3,7):
%   xxxx xxxx 0xxx x110 - Shutdown
%   xxxx xxxx 0xxx 0111 - Switch on
%   xxxx xxxx 0xxx 1111 - Switch on
%   xxxx xxxx 0xxx xx0x - Disable voltage
%   xxxx xxxx 0xxx x01x - Quick stop
%   xxxx xxxx 0xxx 0111 - Disable operation
%   xxxx xxxx 0xxx 1111 - Enable operation
%   xxxx xxxx 1xxx xxxx - Fault reset
%
% Status Word (uint16) (Pg. 29 DSP 402):
%   0 - Ready to switch on
%   1 - Switched on
%   2 - Operation enabled
%   3 - Fault
%   4 - Voltage enabled
%   5 - Quick stop
%   6 - Switch on disabled
%   7 - Warning
%   8 - Manufacturer specific
%   9 - Remote
%   10 - Target reached
%   11 - Internal limit active
%   12...13 - Operation mode specific
%   14...15 - Manufacturer specific
% 
% Device status (Bits 0,1,2,3,5,6):
%   xxxx xxxx x0xx 0000 = Not ready to switch on
%   xxxx xxxx x1xx 0000 = Switch on disabled
%   xxxx xxxx x01x 0001 = Ready to switch on
%   xxxx xxxx x01x 0011 = Switched on
%   xxxx xxxx x01x 0111 = Operation enabled
%   xxxx xxxx x00x 0111 = Quick stop active
%   xxxx xxxx x0xx 1111 = Fault reaction active
%   xxxx xxxx x0xx 1000 = Fault
%
% Modes of Operation (int8) (Pg. 36 of DSP 402):
%   -128...-2 = Reserved
%   -1 = No mode
%   0 = Reserved
%   1 = Profile position mode
%   2 = Velocity (not supported)
%   3 = Profile velocity mode
%   4 = Profile torque mode
%   5 = Reserved
%   6 = Homing mode
%   7 = Interpolated position mode
%   8...127 = Reserved
  
  % Initialize control word to enable operation
  controlWord = uint16(bin2dec('0000000000001111'));
  
  % FAULT -----------------------------------------------------------------
  
  % State Transition 14: FAULT REACTION ACTIVE => FAULT
  
  % State Transition 15: FAULT=>SWITCH ON DISABLED
  if all(bitget(statusWord, [7 4 3 2 1]) == [0 1 0 0 0])
    % Set control word to fault reset (xxxx xxxx 1xxx xxxx)
    controlWord = bitset(controlWord, 8, 1);
  end % if
  
  % POWER DISABLED --------------------------------------------------------
  
  % State Transition 0: START => NOT READY TO SWITCH ON
  
  % State Transition 1: NOT READY TO SWITCH ON => SWITCH ON DISABLED
  
  % State Transition 2: SWITCH ON DISABLED => READY TO SWITCH ON
  if all(bitget(statusWord, [7 4 3 2 1]) == [1 0 0 0 0])
    % Set control word to shutdown (xxxx xxxx 0xxx x110)
    controlWord = bitset(controlWord, 1, 0);
    controlWord = bitset(controlWord, 2, 1);
    controlWord = bitset(controlWord, 3, 1);
    controlWord = bitset(controlWord, 8, 0);
  end % if

  % State Transition 3: READY TO SWITCH ON => SWITCHED ON
  if all(bitget(statusWord, [7 6 4 3 2 1]) == [0 1 0 0 0 1])
    % Set control word to switch on (xxxx xxxx 0xxx 0111)
    controlWord = bitset(controlWord, 1, 1);
    controlWord = bitset(controlWord, 2, 1);
    controlWord = bitset(controlWord, 3, 1);
    controlWord = bitset(controlWord, 4, 0);
    controlWord = bitset(controlWord, 8, 0);
  end % if
  
  % POWER ENABLED ---------------------------------------------------------
  
  % State Transition 4: SWITCHED ON => OPERATION ENABLE
  if all(bitget(statusWord, [7 6 4 3 2 1]) == [0 1 0 0 1 1])
    % Set control word to enable operation (xxxx xxxx 0xxx 1111)
    controlWord = bitset(controlWord, 1, 1);
    controlWord = bitset(controlWord, 2, 1);
    controlWord = bitset(controlWord, 3, 1);
    controlWord = bitset(controlWord, 4, 1);
    controlWord = bitset(controlWord, 8, 0);
  end % if
end % elmoStateMachine

== matlab function RealTimeLibrary/Battery Management System/ADC to Amperage MATLAB Function ==
  data: adcValue input; A output
function A = adcToAmperage(adcValue) %#codegen
%ADCTOAMPERAGE Convert ADC value to amperage.
%
% Description:
%   The current transducer is connected to the AUXn input channels on the
%   battery monitor chip. In order to get a current reading we have to
%     - Convert the returned ADC value to voltage given the battery
%     monitor specifications
%     - Convert voltage to amperage given the current transducer
%     specifications
%
% Specifications:
%   - Battery Monitor: bq76pl455a-q1
%     - http://www.ti.com/lit/ds/symlink/bq76pl455a-q1.pdf
%     - V_REF = 2.5V
%     - V_AUX = (2*V_REF)/65535*READ_ADC_VALUE
%
%   - Current Transducer: ACS770KCB-150B-PFF-T
%     - https://en.wikipedia.org/wiki/Voltage_divider
%     - sensitivity = 13.3mV/A

% Copyright 2017 Mikhail S. Jones

  sensitivity = 13.3/1000;
  V_ref = 2.5;
  V = (2.*V_ref)./65535.*adcValue;
  A = (V - 2.5)./sensitivity;
end % convertToAmperage

== matlab function RealTimeLibrary/Battery Management System/ADC to Voltage MATLAB Function ==
  data: adcValue input; V output
function V = adcToVoltage(adcValue) %#codegen
%ADCTOVOLTAGE Convert ADC value to voltage.
% 
% Description:
%   The voltage taps are connected to the VSENSE input channels on the
%   battery monitor chip. In order to get a voltage reading we have to
%     - Convert the returned ADC value to voltage given the battery
%     monitor specifications
%
% Specifications:
%   - Battery Monitor: bq76pl455a-q1
%     - http://www.ti.com/lit/ds/symlink/bq76pl455a-q1.pdf
%     - V_REF = 2.5V
%     - V_AUX = (2*V_REF)/65535*READ_ADC_VALUE

% Copyright 2017 Mikhail S. Jones

  V_ref = 2.5;
  V = (2.*V_ref)./65535.*adcValue;
end % adcToVoltage

== matlab function RealTimeLibrary/Battery Management System/ADC to Celcius MATLAB Function ==
  data: adcValue input; C output
function C = adcToCelcius(adcValue) %#codegen
%ADCTOCELCIUS Convert ADC value to Celcius.
%
% Description:
%   The thermistors are connected to the AUXn input channels on the battery
%   monitor chip. In order to get a temperature reading we have to
%     - Convert the returned ADC value to voltage given the battery
%     monitor specifications
%     - Convert voltage to resistance given the voltage divider circuit
%     on the BMS board
%    - Convert resistance to temperature given the thermistor
%    specifications
%
% Specifications:
%   - Battery Monitor: bq76pl455a-q1
%     - http://www.ti.com/lit/ds/symlink/bq76pl455a-q1.pdf
%     - V_REF = 2.5V
%     - V_AUX = (2*V_REF)/65535*READ_ADC_VALUE
%
%   - Voltage Divider
%     - https://en.wikipedia.org/wiki/Voltage_divider
%     - R_THERM = 10000*(5/V_AUX - 1)
%
%   - Thermistor: BC2647-ND
%     - http://www.vishay.com/docs/29078/ntcle413.pdf
%     - https://en.wikipedia.org/wiki/Thermistor
%     - B = 3435, R0 = 10k, T0 = 298.15 and Rinf = 0.099191
%     - T = B/ln(R/Rinf)

% Copyright 2017 Mikhail S. Jones
  
  V_ref = 2.5;
  V = (2.*V_ref)./65535.*adcValue;
  R = 10000.*(5./V - 1);
  K = 3435./log(R./0.099191);
  C = K - 273.15;
end % adcToCelcius

== matlab function RealTimeLibrary/Gold Twitter/Millivolt to Celcius MATLAB Function ==
  data: mV input; C output
function C = millivoltToCelcius(mV) %#codegen
%MILLIVOLTTOCELCIUS Convert millivolt to Celcius.
%
% Description:
%   The thermistors are connected to the AUXn input channels on the battery
%   monitor chip. In order to get a temperature reading we have to
%     - Convert voltage to resistance given the voltage divider circuit on
%     the twitter breakout board
%     - Convert resistance to temperature given the thermistor
%     specifications
%
% Specifications:
%   - Voltage Divider:
%     - https://en.wikipedia.org/wiki/Voltage_divider
%
%   - Thermistor: 
%     - https://en.wikipedia.org/wiki/Thermistor
%     - B = 3974, R0 = 33k, T0 = 298.15 and Rinf = 0.0536862
%     - T = B/ln(R/Rinf)

% Copyright 2017 Mikhail S. Jones

  V = mV/1000;
  R_tot = (33000.*V./5)./(1 - (V./5));
  R_th = (R_tot*3740)./(3740 - R_tot);
  K = 3974./log(R_th./0.0536862);
  C = K - 273.15;
end % millivoltToCelcius
